simulink subsystem "EG_EngineDynamic"  (R2025a)
settings: Solver=VariableStepAuto  StartTime=0.0  StopTime=10.0  RelTol=1e-3
undefined symbols (not defined in the file): EG_BladesInteria_P, EG_EngineGain_P, EG_EngineTorqueMax_P, EG_HubInteria_P, EG_TailRotorGearRatio_P, EG_TauEngine10Coeff_P, EG_TauEngine11Coeff_P, EG_TauEngine20Coeff_P, EG_TauEngine21Coeff_P, EG_TurbinInteria_P
libraries: slpidlib x1
settings Model: DataDictionary=Engine.sldd  EnableAccessToBaseWorkspace=off  DefaultTestHarness=EG_EngineDynamic_Harness  Creator=LAPTOP  LastModifiedBy=LAPTOP

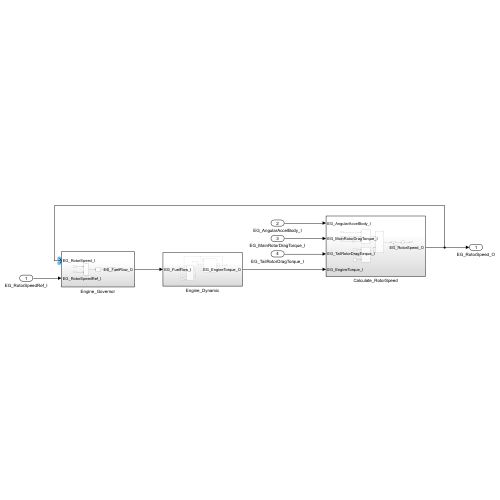
[thumbnail: Simulink's stored preview of the top-level diagram]
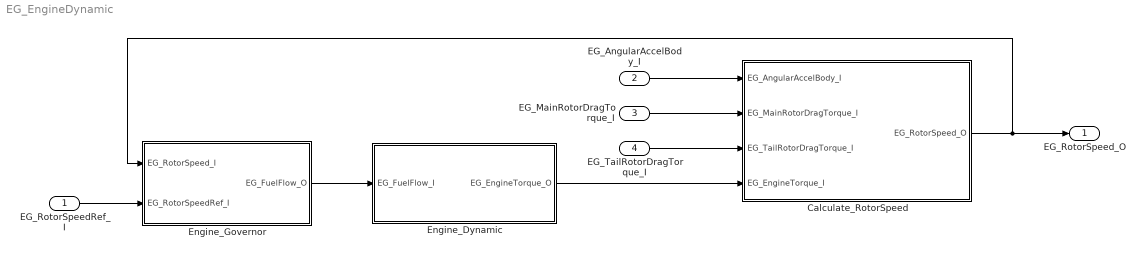
== system EG_EngineDynamic ==
  EG_RotorSpeedRef_I : Inport
  EG_AngularAccelBody_I : Inport  Port=2
  EG_MainRotorDragTorque_I : Inport  Port=3
  EG_TailRotorDragTorque_I : Inport  Port=4
  Calculate_RotorSpeed : Subsystem
  Engine_Dynamic : Subsystem
  Engine_Governor : Subsystem
  EG_RotorSpeed_O : Outport
  wires:
  Engine_Dynamic/1(EG_EngineTorque_O) -> Calculate_RotorSpeed/4(EG_EngineTorque_I)
  Engine_Governor/1(EG_FuelFlow_O) -> Engine_Dynamic/1(EG_FuelFlow_I)
  Calculate_RotorSpeed/1(EG_RotorSpeed_O) -> Engine_Governor/1(EG_RotorSpeed_I), EG_RotorSpeed_O/1
  EG_RotorSpeedRef_I/1 -> Engine_Governor/2(EG_RotorSpeedRef_I)
  EG_TailRotorDragTorque_I/1 -> Calculate_RotorSpeed/3(EG_TailRotorDragTorque_I)
  EG_MainRotorDragTorque_I/1 -> Calculate_RotorSpeed/2(EG_MainRotorDragTorque_I)
  EG_AngularAccelBody_I/1 -> Calculate_RotorSpeed/1(EG_AngularAccelBody_I)

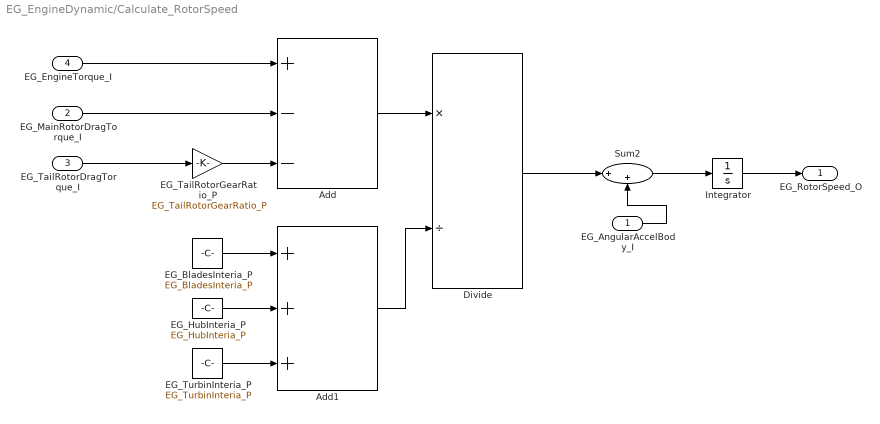
== system EG_EngineDynamic/Calculate_RotorSpeed ==
  EG_AngularAccelBody_I : Inport
  EG_MainRotorDragTorque_I : Inport  Port=2
  EG_TailRotorDragTorque_I : Inport  Port=3
  EG_EngineTorque_I : Inport  Port=4
  Add : Sum  Inputs=+--
  Add1 : Sum  Inputs=+++
  Divide : Product  Inputs=*/
  EG_BladesInteria_P : Constant  Value=EG_BladesInteria_P
  EG_HubInteria_P : Constant  Value=EG_HubInteria_P
  EG_TailRotorGearRatio_P : Gain  Gain=EG_TailRotorGearRatio_P
  EG_TurbinInteria_P : Constant  Value=EG_TurbinInteria_P
  Integrator : Integrator
  Sum2 : Sum  Inputs=|++
  EG_RotorSpeed_O : Outport
  wires:
  EG_TailRotorDragTorque_I/1 -> EG_TailRotorGearRatio_P/1
  EG_BladesInteria_P/1 -> Add1/1
  EG_HubInteria_P/1 -> Add1/2
  EG_TurbinInteria_P/1 -> Add1/3
  EG_EngineTorque_I/1 -> Add/1
  EG_MainRotorDragTorque_I/1 -> Add/2
  EG_TailRotorGearRatio_P/1 -> Add/3
  Add/1 -> Divide/1
  Add1/1 -> Divide/2
  Divide/1 -> Sum2/1
  Sum2/1 -> Integrator/1
  Integrator/1 -> EG_RotorSpeed_O/1
  EG_AngularAccelBody_I/1 -> Sum2/2

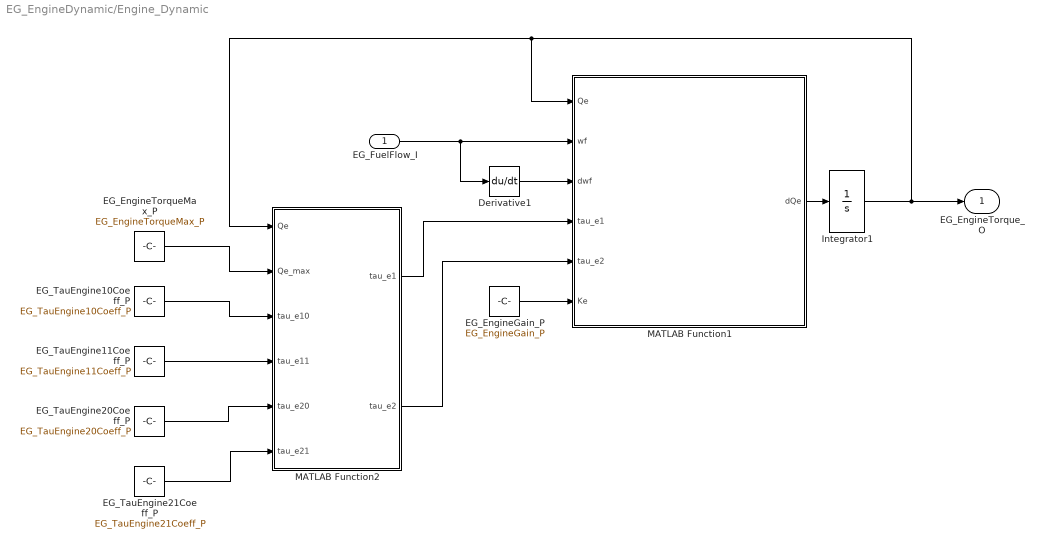
== system EG_EngineDynamic/Engine_Dynamic ==
  EG_FuelFlow_I : Inport
  Derivative1 : Derivative
  EG_EngineGain_P : Constant  Value=EG_EngineGain_P
  EG_EngineTorqueMax_P : Constant  Value=EG_EngineTorqueMax_P
  EG_TauEngine10Coeff_P : Constant  Value=EG_TauEngine10Coeff_P
  EG_TauEngine11Coeff_P : Constant  Value=EG_TauEngine11Coeff_P
  EG_TauEngine20Coeff_P : Constant  Value=EG_TauEngine20Coeff_P
  EG_TauEngine21Coeff_P : Constant  Value=EG_TauEngine21Coeff_P
  Integrator1 : Integrator
  MATLAB Function1 : MATLAB Function  TreatAsAtomicUnit=on
  MATLAB Function2 : MATLAB Function  TreatAsAtomicUnit=on
  EG_EngineTorque_O : Outport
  wires:
  Integrator1/1 -> MATLAB Function2/1(Qe), MATLAB Function1/1(Qe), EG_EngineTorque_O/1
  MATLAB Function1/1(dQe) -> Integrator1/1
  EG_EngineGain_P/1 -> MATLAB Function1/6(Ke)
  EG_FuelFlow_I/1 -> MATLAB Function1/2(wf), Derivative1/1
  Derivative1/1 -> MATLAB Function1/3(dwf)
  MATLAB Function2/1(tau_e1) -> MATLAB Function1/4(tau_e1)
  MATLAB Function2/2(tau_e2) -> MATLAB Function1/5(tau_e2)
  EG_EngineTorqueMax_P/1 -> MATLAB Function2/2(Qe_max)
  EG_TauEngine10Coeff_P/1 -> MATLAB Function2/3(tau_e10)
  EG_TauEngine11Coeff_P/1 -> MATLAB Function2/4(tau_e11)
  EG_TauEngine20Coeff_P/1 -> MATLAB Function2/5(tau_e20)
  EG_TauEngine21Coeff_P/1 -> MATLAB Function2/6(tau_e21)

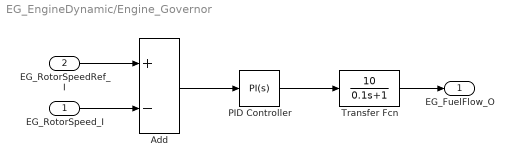
== system EG_EngineDynamic/Engine_Governor ==
  EG_RotorSpeed_I : Inport
  EG_RotorSpeedRef_I : Inport  Port=2
  Add : Sum  Inputs=+-
  PID Controller : slpidlib/PID Controller  Controller=PI  Form=Ideal  TimeDomain=Continuous-time  UseExternalTs=off  SampleTime=-1  IntegratorMethod=Forward Euler  FilterMethod=Forward Euler  ControllerParametersSource=internal  P=0.025  I=10  UseKiTs=off  D=0  UseExternalDerivativeSource=off  N=100  UseFilter=on  TunerSelectOption=Transfer Function Based (PID Tuner App)  InitialConditionSource=internal  InitialConditionForIntegrator=0  InitialConditionForFilter=0  DifferentiatorICPrevScaledInput=0  ExternalReset=none  TrackingMode=off  Kt=1  LimitOutput=off  SatLimitsSource=internal  UpperSaturationLimit=inf  LowerSaturationLimit=-inf  LinearizeAsGain=on  AntiWindupMode=none  Kb=1  LimitIntegrator=off  UpperIntegratorSaturationLimit=inf  LowerIntegratorSaturationLimit=-inf  POutMin=[]  POutMax=[]  IOutMin=[]  IOutMax=[]  DOutMin=[]  DOutMax=[]  NOutMin=[]  NOutMax=[]  SumOutMin=[]  SumOutMax=[]  SaturationOutMin=[]  SaturationOutMax=[]  PParamMin=[]  PParamMax=[]  IParamMin=[]  IParamMax=[]  DParamMin=[]  DParamMax=[]  NParamMin=[]  NParamMax=[]  KbParamMin=[]  KbParamMax=[]  KtParamMin=[]  KtParamMax=[]  KbOutMin=[]  KbOutMax=[]  KtOutMin=[]  KtOutMax=[]  IntegratorOutMin=[]  IntegratorOutMax=[]  FilterOutMin=[]  FilterOutMax=[]  SumI1OutMin=[]  SumI1OutMax=[]  SumI2OutMin=[]  SumI2OutMax=[]  SumI3OutMin=[]  SumI3OutMax=[]  SumI4OutMin=[]  SumI4OutMax=[]  SumDOutMin=[]  SumDOutMax=[]  DifferentiatorOutMin=[]  DifferentiatorOutMax=[]  FilterDiffOutCoefMin=[]  FilterDiffOutCoefMax=[]  ReciprocalOutMin=[]  ReciprocalOutMax=[]  SumDenOutMin=[]  SumDenOutMax=[]  SumNumOutMin=[]  SumNumOutMax=[]  DivideOutMin=[]  DivideOutMax=[]  UdiffTsProdOutMin=[]  UdiffTsProdOutMax=[]  NTsProdOutMin=[]  NTsProdOutMax=[]  UintegralTsProdOutMin=[]  UintegralTsProdOutMax=[]  UngainTsProdOutMin=[]  UngainTsProdOutMax=[]  ClampingZeroOutDataTypeStr=Inherit: Inherit via back propagation  ClampingZeroOutMin=[]  ClampingZeroOutMax=[]  FilterDenConstantOutDataTypeStr=Inherit: Inherit via back propagation  FilterDenConstantOutMin=[]  FilterDenConstantOutMax=[]  PCopyOutDataTypeStr=Inherit: Inherit via back propagation  PCopyOutMin=[]  PCopyOutMax=[]  NCopyOutDataTypeStr=Inherit: Inherit via back propagation  NCopyOutMin=[]  NCopyOutMax=[]  IntegratorContinuousStateAttributes=''  IntegratorStateMustResolveToSignalObject=off  IntegratorRTWStateStorageClass=Auto  FilterContinuousStateAttributes=''  FilterStateMustResolveToSignalObject=off  FilterRTWStateStorageClass=Auto  ParallelPVariant=Passthrough  IdealPVariant=InternalParameters  IVariant=InternalParameters  DVariant=Disabled  IntegratorVariant=Continuous  SatVariant=Disabled  AWVariant=Passthrough  PCopyVariant=Disabled  TRVariant=Disabled  FdbkBlocksVariant=Forward  IdealPFdbkVariant=Disabled  SatFdbkVariant=Disabled  DerivativeFilterVariant=Disabled  NVariant=Disabled  NCopyVariant=Disabled_SignalSpec  FilterICVariant=Disabled  IntegratorICVariant=InternalICs  ExternalResetVariant=Disabled  TRSumVariant=Passthrough  SumFdbkVariant=Disabled  SumVariant=Sum_PI  TsampFilterVariant=InternalTs  TsampNgainVariant=Passthrough  TsampIntegralVariant=Disabled_SignalSpec  ExternalSaturationOutDataTypeStr=Inherit: Same as second input  DerivativeSourceVariant=Disabled  PreIntVariant=InternalPreInt
  Transfer Fcn : TransferFcn  Numerator=[10]  Denominator=[0.1 1]
  EG_FuelFlow_O : Outport
  wires:
  EG_RotorSpeed_I/1 -> Add/2
  EG_RotorSpeedRef_I/1 -> Add/1
  Transfer Fcn/1 -> EG_FuelFlow_O/1
  Add/1 -> PID Controller/1
  PID Controller/1 -> Transfer Fcn/1

== matlab function EG_EngineDynamic/Engine_Dynamic/MATLAB Function1 ==
  data: Qe input; dQe output; wf input; dwf input; tau_e1 input; tau_e2 input; Ke input
function dQe = engine_torque_dynamics(Qe, wf, dwf, tau_e1, tau_e2, Ke)
% MATLAB Function tính toán đạo hàm mô-men xoắn động cơ
% Dựa trên mô hình động cơ bậc 2 trong tài liệu
%
% Inputs:
%   Qe     : Mô-men xoắn động cơ hiện tại (Phản hồi từ Integrator)
%   wf     : Lưu lượng nhiên liệu (Fuel flow)
%   dwf    : Đạo hàm lưu lượng nhiên liệu (d/dt wf)
%   tau_e1 : Hằng số thời gian động cơ 1 (từ khối tính toán tau)
%   tau_e2 : Hằng số thời gian động cơ 2 (từ khối tính toán tau)
%   Ke     : Hệ số tăng của động cơ (Engine Gain)
%
% Output:
%   dQe    : Đạo hàm mô-men xoắn (Qe_dot) -> Đưa vào Integrator

    % Triển khai công thức:
    % Qe_dot = (1/tau_e2) * [Ke*wf + Ke*tau_e1*dwf - Qe]
    
    dQe = (1/tau_e2) * (Ke * wf + Ke * tau_e1 * dwf - Qe);

end

== matlab function EG_EngineDynamic/Engine_Dynamic/MATLAB Function2 ==
  data: Qe input; tau_e1 output; Qe_max input; tau_e2 output; tau_e10 input; tau_e11 input; tau_e20 input; tau_e21 input
function [tau_e1, tau_e2] = calc_tau(Qe, Qe_max, tau_e10, tau_e11, tau_e20, tau_e21)
    % Qe_bar là tỷ lệ % so với Qe_max
    Qe_bar = Qe / Qe_max;
    
    tau_e1 = tau_e10 + tau_e11 * Qe_bar;
    tau_e2 = tau_e20 + tau_e21 * Qe_bar;
end
